simulink model "inverse_kinematics_model"  (R2025a)
settings: Solver=FixedStepAuto  StartTime=0.0  StopTime=40  FixedStep=0.001  RelTol=1e-3  EnableMultiTasking=on
libraries: robotmaniplib x4
settings Model: SILPILModeSetting=veronly  ExtModeTrigDuration=2  Creator=jonas  LastModifiedBy=zafi
settings SolverCC: AllowMultiTaskInputOutput=on  ConcurrentTasks=on
settings OptimizationCC: DefaultUnderspecifiedDataType=single  EnhancedBackFolding=on  PassReuseOutputArgsAs=Individual arguments  ZeroExternalMemoryAtStartup=off  ZeroInternalMemoryAtStartup=off  EfficientFloat2IntCast=on  MaxStackSize=64  SimCompilerOptimization=on  OptimizeBlockOrder=speed  DifferentSizesBufferReuse=on  OptimizationCustomize=off  EfficientTunableParamExpr=on
settings DebuggingCC: ParameterTunabilityLossMsg=error
settings HardwareCC: ProdBitPerInt=16.0  ProdBitPerPointer=16.0  ProdBitPerSizeT=16.0  ProdBitPerPtrDiffT=16.0  ProdLargestAtomicFloat=None  ProdWordSize=8.0  ProdHWDeviceType=Atmel->AVR
settings ModelReferenceCC: EnableParallelModelReferenceBuilds=on  ModelReferenceMinAlgLoopOccurrences=on
settings SFSimCC: MATLABDynamicMemAllocThreshold=32000.0  SimTargetLang=C++  SimDLTargetLibrary=mkl-dnn
settings RTWCC: SystemTargetFile=ert.tlc  HardwareBoard=Arduino Mega 2560  TemplateMakefile=ert_default_tmf  Toolchain=Arduino AVR  BuildConfiguration=Faster Runs  GPUComputeCapability=3.5  Description=Embedded Coder
settings CodeAppCC: ForceParamTrailComments=on  IgnoreCustomStorageClasses=off  OperatorAnnotations=on  SimulinkDataObjDesc=on  SFDataObjDesc=on  InsertBlockDesc=on
settings ERTTargetCC: ExtModeTransport=3.0  ExtModeAutomaticAllocSize=off  ExtModeStaticAllocSize=2048.0  InlinedParameterPlacement=Hierarchical  DynamicArrayContainerType=coder::array  SupportContinuousTime=on  SupportVariableSizeSignals=on

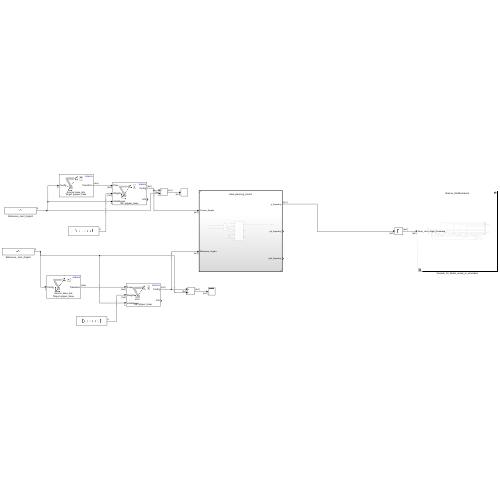
[thumbnail: Simulink's stored preview of the top-level diagram]
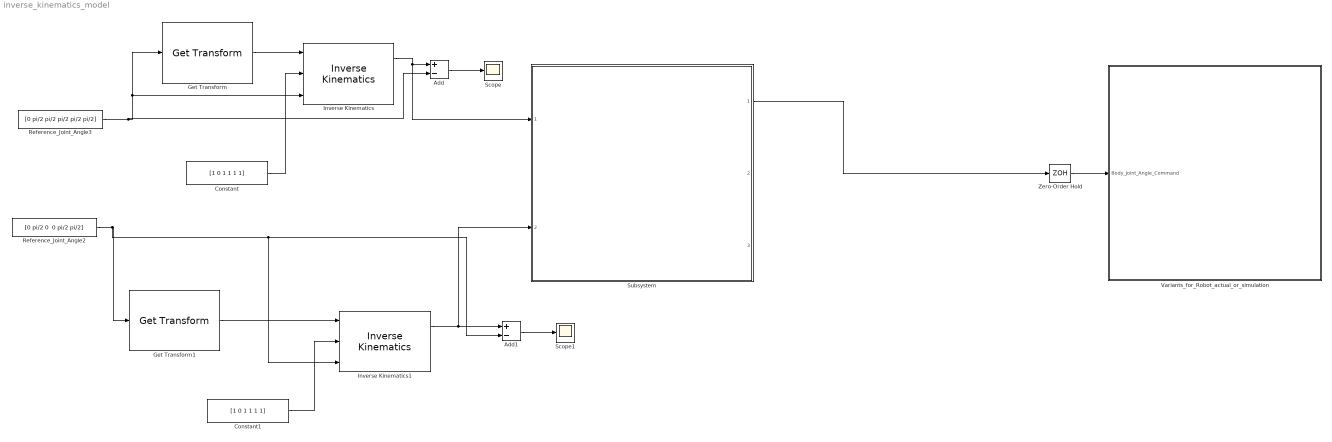
== system inverse_kinematics_model ==
  Add : Sum  Inputs=+-
  Add1 : Sum  Inputs=+-
  Constant : Constant  Value=[1 0 1 1 1 1]
  Constant1 : Constant  Value=[1 0 1 1 1 1]
  Get Transform : robotmaniplib/Get Transform  RigidBodyTree=braccio  SourceBody=base_link  TargetBody=gripper_base  SimulateUsing=Interpreted execution
  Get Transform1 : robotmaniplib/Get Transform  RigidBodyTree=braccio  SourceBody=base_link  TargetBody=gripper_base  SimulateUsing=Interpreted execution
  Inverse Kinematics : robotmaniplib/Inverse Kinematics  RigidBodyTree=braccio  EndEffector=gripper_base  ShowInfo=on  SolverName=BFGS Gradient Projection  EnforceJointLimits=on  MaxIterations=1500  MaxTime=10  GradientTolerance=1e-7  SolutionTolerance=1e-6  StepTolerance=1e-14  ConstraintTolerance=1e-6  ErrorChangeTolerance=1e-12  UseErrorDamping=on  DampingBias=0.0025  SimulateUsing=Interpreted execution
  Inverse Kinematics1 : robotmaniplib/Inverse Kinematics  RigidBodyTree=braccio  EndEffector=gripper_base  ShowInfo=on  SolverName=BFGS Gradient Projection  EnforceJointLimits=on  MaxIterations=1500  MaxTime=10  GradientTolerance=1e-7  SolutionTolerance=1e-6  StepTolerance=1e-14  ConstraintTolerance=1e-6  ErrorChangeTolerance=1e-12  UseErrorDamping=on  DampingBias=0.0025  SimulateUsing=Interpreted execution
  Reference_Joint_Angle2 : Constant  Value="[0 pi/2 0  0 pi/2 pi/2]"
  Reference_Joint_Angle3 : Constant  Value=[0 pi/2 pi/2 pi/2 pi/2 pi/2]
  Scope : Scope
      settings: ActiveDisplayYMinimum=-112.61641460522705  ActiveDisplayYMaximum=45.897286494747739  DataLoggingVariableName=ScopeData3
  Scope1 : Scope
      settings: ActiveDisplayYMinimum=-0.33460521243595137  ActiveDisplayYMaximum=0.044387183533202416  DataLoggingVariableName=ScopeData4
  Subsystem : Subsystem  TreatAsAtomicUnit=on  ReferencedSubsystem=robot_planning_control
  Variants_for_Robot_actual_or_simulation : Subsystem  TreatAsAtomicUnit=on  Variant=on  VariantChoicesSpecifier={'Braccio_Arduino', 'Braccio_SimMechanics'}  VariantControlMode=label  VariantControl=Choice  LabelModeActiveChoice=Braccio_SimMechanics
  Zero-Order Hold : ZeroOrderHold  SampleTime=-1
  wires:
  Zero-Order Hold/1 -> Variants_for_Robot_actual_or_simulation/1(Body_Joint_Angle_Command)
  Subsystem/1 -> Zero-Order Hold/1
  Reference_Joint_Angle3/1 -> Add/2, Inverse Kinematics/3, Get Transform/1
  Get Transform/1 -> Inverse Kinematics/1
  Constant/1 -> Inverse Kinematics/2
  Inverse Kinematics/1 -> Subsystem/1, Add/1
  Add/1 -> Scope/1
  Get Transform1/1 -> Inverse Kinematics1/1
  Add1/1 -> Scope1/1
  Inverse Kinematics1/1 -> Subsystem/2, Add1/1
  Constant1/1 -> Inverse Kinematics1/2
  Reference_Joint_Angle2/1 -> Inverse Kinematics1/3, Add1/2, Get Transform1/1

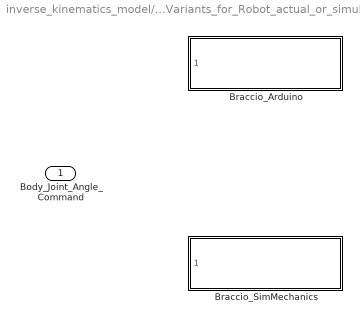
== system inverse_kinematics_model/Variants_for_Robot_actual_or_simulation ==
  Body_Joint_Angle_Command : Inport
  Braccio_Arduino : Subsystem  TreatAsAtomicUnit=on  VariantControl=Braccio_Arduino  ReferencedSubsystem=Braccio_Arduino
  Braccio_SimMechanics : Subsystem  TreatAsAtomicUnit=on  VariantControl=Braccio_SimMechanics  ReferencedSubsystem=Braccio_SimMechanics
